simulink subsystem "IMU3"  (R2021a)
settings: Solver=VariableStepAuto  StartTime=0.0  StopTime=10.0  RelTol=1e-3
undefined symbols (not defined in the file): imu3, Ts
libraries: simulink x8, dspsrcs4 x3, dspmtrx3 x2
settings Model: Creator=Laura  LastModifiedBy=Laura

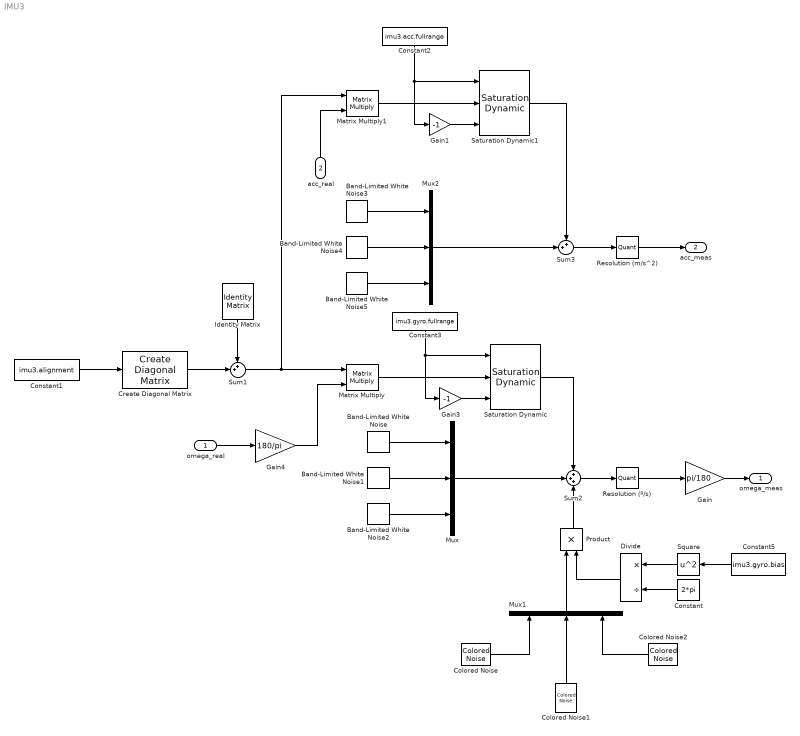
== system IMU3 ==
  omega_real : Inport
  acc_real : Inport  Port=2
  Band-Limited White Noise : simulink/Sources/Band-Limited White Noise  Cov=imu3.gyro.noisepower(1)  Ts=Ts  seed=[234234111]
  Band-Limited White Noise1 : simulink/Sources/Band-Limited White Noise  Cov=imu3.gyro.noisepower(2)  Ts=Ts  seed=[567380]
  Band-Limited White Noise2 : simulink/Sources/Band-Limited White Noise  Cov=imu3.gyro.noisepower(3)  Ts=Ts  seed=[3256]
  Band-Limited White Noise3 : simulink/Sources/Band-Limited White Noise  Cov=imu3.acc.noisepower(1)  Ts=Ts  seed=[32323556]
  Band-Limited White Noise4 : simulink/Sources/Band-Limited White Noise  Cov=imu3.acc.noisepower(2)  Ts=Ts  seed=[238641]
  Band-Limited White Noise5 : simulink/Sources/Band-Limited White Noise  Cov=imu3.acc.noisepower(3)  Ts=Ts  seed=[23341231]
  Colored Noise : dspsrcs4/Colored Noise  Color=pink  InverseFrequencyPower=1  BoundedOutput=off  NumChannels=1  OutputDataType=double  SamplesPerFrame=1  SampleTime=Ts  RandomStream=mt19937ar with seed  Seed=12237  SimulateUsing=Interpreted execution
      settings: SourceProductBaseCode=DS
  Colored Noise1 : dspsrcs4/Colored Noise  Color=pink  InverseFrequencyPower=1  BoundedOutput=off  NumChannels=1  OutputDataType=double  SamplesPerFrame=1  SampleTime=Ts  RandomStream=mt19937ar with seed  Seed=76372  SimulateUsing=Interpreted execution
      settings: SourceProductBaseCode=DS
  Colored Noise2 : dspsrcs4/Colored Noise  Color=pink  InverseFrequencyPower=1  BoundedOutput=off  NumChannels=1  OutputDataType=double  SamplesPerFrame=1  SampleTime=Ts  RandomStream=mt19937ar with seed  Seed=3755  SimulateUsing=Interpreted execution
      settings: SourceProductBaseCode=DS
  Constant : Constant  Value=2*pi
  Constant1 : Constant  Value=imu3.alignment
  Constant2 : Constant  Value=imu3.acc.fullrange
  Constant3 : Constant  Value=imu3.gyro.fullrange
  Constant5 : Constant  Value=imu3.gyro.bias
  Create Diagonal Matrix : dspmtrx3/Create Diagonal Matrix
      settings: SourceProductBaseCode=DS
  Divide : Product  Inputs=*/
  Gain : Gain  Gain=pi/180
  Gain1 : Gain  Gain=-1
  Gain3 : Gain  Gain=-1
  Gain4 : Gain  Gain=180/pi
  Identity Matrix : dspmtrx3/Identity Matrix  Inherit=off  N=3  Ts=1  dataType=double  isSigned=on  wordLen=16  udDataType=sfix(16)  fracBitsMode=Best precision  numFracBits=15  OutDataTypeStr=double  LastOutDataTypeStr=double
  Matrix Multiply : Product  Multiplication=Matrix(*)
  Matrix Multiply1 : Product  Multiplication=Matrix(*)
  Mux : Mux  Inputs=3
  Mux1 : Mux  Inputs=3
  Mux2 : Mux  Inputs=3
  Product : Product
  Resolution (m/s^2) : Quantizer  QuantizationInterval=imu3.acc.quantization  LinearizeAsGain=off
  Resolution (º/s) : Quantizer  QuantizationInterval=imu3.gyro.quantization  LinearizeAsGain=off
  Saturation Dynamic : simulink/Discontinuities/Saturation Dynamic  OutMin=[]  OutMax=[]  OutDataTypeStr=Inherit: Same as second input  OutDataType=fixdt(1, 16)  OutScaling=2^-10  DoSatur=off
  Saturation Dynamic1 : simulink/Discontinuities/Saturation Dynamic  OutMin=[]  OutMax=[]  OutDataTypeStr=Inherit: Same as second input  OutDataType=fixdt(1, 16)  OutScaling=2^-10  DoSatur=off
  Square : Math  Operator=square  SaturateOnIntegerOverflow=on
  Sum1 : Sum  Inputs=++|
  Sum2 : Sum  Inputs=+++
  Sum3 : Sum  Inputs=++|
  omega_meas : Outport  SampleTime=Ts
  acc_meas : Outport  Port=2  SampleTime=Ts
  wires:
  Band-Limited White Noise3/1 -> Mux2/1
  Band-Limited White Noise5/1 -> Mux2/3
  Mux/1 -> Sum2/2
  Square/1 -> Divide/1
  Gain/1 -> omega_meas/1
  Constant/1 -> Divide/2
  Gain4/1 -> Matrix Multiply/2
  Identity Matrix/1 -> Sum1/1
  Divide/1 -> Product/2
  Band-Limited White Noise1/1 -> Mux/2
  Mux1/1 -> Product/1
  Product/1 -> Sum2/3
  Saturation Dynamic/1 -> Sum2/1
  Matrix Multiply/1 -> Saturation Dynamic/2
  Gain3/1 -> Saturation Dynamic/3
  omega_real/1 -> Gain4/1
  Band-Limited White Noise/1 -> Mux/1
  Sum2/1 -> Resolution (º/s)/1
  Band-Limited White Noise2/1 -> Mux/3
  Sum1/1 -> Matrix Multiply/1, Matrix Multiply1/1
  Matrix Multiply1/1 -> Saturation Dynamic1/2
  Constant3/1 -> Saturation Dynamic/1, Gain3/1
  Sum3/1 -> Resolution (m/s^2)/1
  Colored Noise1/1 -> Mux1/2
  Create Diagonal Matrix/1 -> Sum1/2
  Constant2/1 -> Gain1/1, Saturation Dynamic1/1
  Constant1/1 -> Create Diagonal Matrix/1
  Colored Noise2/1 -> Mux1/3
  Resolution (m/s^2)/1 -> acc_meas/1
  Mux2/1 -> Sum3/2
  Resolution (º/s)/1 -> Gain/1
  Gain1/1 -> Saturation Dynamic1/3
  Colored Noise/1 -> Mux1/1
  Band-Limited White Noise4/1 -> Mux2/2
  Saturation Dynamic1/1 -> Sum3/1
  acc_real/1 -> Matrix Multiply1/2
  Constant5/1 -> Square/1
